simulink model "Robot_Leg_Kneel"  (R2025b)
settings: Solver=VariableStepAuto  StartTime=0.0  StopTime=20  RelTol=0.01  AbsTol=0.01  EnableMultiTasking=on
undefined symbols (not defined in the file): X, Y, Z
libraries: sm_lib x50, nesl_utility x37
(part 3 of 4)

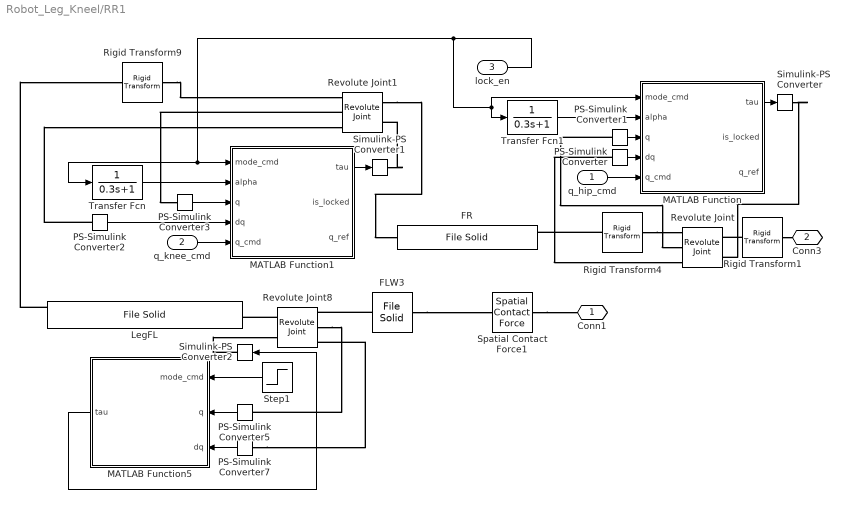
== system Robot_Leg_Kneel/RR1 ==
  q_hip_cmd : Inport
  q_knee_cmd : Inport  Port=2
  lock_en : Inport  Port=3
  FLW3 : sm_lib/Body Elements/File Solid  ExtGeomFileName=Cheng Shin C-166-1.stp  UnitType=FromFile  ExtGeomFileUnits=m  StepReaderType=HEX  ExportConvexHullGeometry=on  InertiaType=CalculateFromGeometry  BasedOnType=Density  Density=400  DensityUnits=kg/m^3  Mass=1  MassUnits=kg  CenterOfMass=[0 0 0]  CenterOfMassUnits=m  MomentsOfInertia=[1 1 1]  MomentsOfInertiaUnits=kg*m^2  ProductsOfInertia=[0 0 0]  ProductsOfInertiaUnits=kg*m^2  GraphicType=FromGeometry  MarkerShape=Sphere  MarkerSize=10  GraphicVisPropType=AdvancedVisualProperties  GraphicDiffuseColor=[0.1 0.1 0.1]  GraphicOpacity=1  GraphicSpecularColor=[0.2 0.2 0.2 1.0]  GraphicAmbientColor=[0.05 0.05 0.05 1.0]  GraphicEmissiveColor=[0.0 0.0 0.0 1.0]  GraphicShininess=10  DoExposeReferenceFrame=off  SerializedFrames=|
      | <Frames>
      | 
      |   <Frame>
      |     <Id>Frame1</Id>
      |     <Value>
      |       <Name>F1</Name>
      |       <Origin>
      |         <Source>GeometricFeature</Source>
      |         <FeatureName>toroidal surface 99</FeatureName>
      |       </Origin>
      |       <PrimaryAxis>
      |         <DefinedDirection>+Z</DefinedDirection>
      |         <Source>ReferenceFrame</Source>
      |         <SourceDirection>+Z</SourceDirection>
      |         <FeatureName></FeatureName>
      |       </PrimaryAxis>
      |       <SecondaryAxis>
      |         <DefinedDirection>+X</DefinedDirection>
      |         <Source>ReferenceFrame</Source>
      |         <SourceDirection>+X</SourceDirection>
      |         <FeatureName></FeatureName>
      |       </SecondaryAxis>
      |     </Value>
      |   </Frame>
      | 
      | </Frames>
  FR : sm_lib/Body Elements/File Solid  ExtGeomFileName=haut patte D.STEP  UnitType=FromFile  ExtGeomFileUnits=m  StepReaderType=HEX  ExportConvexHullGeometry=on  InertiaType=CalculateFromGeometry  BasedOnType=Density  Density=800  DensityUnits=kg/m^3  Mass=1  MassUnits=kg  CenterOfMass=[0 0 0]  CenterOfMassUnits=m  MomentsOfInertia=[1 1 1]  MomentsOfInertiaUnits=kg*m^2  ProductsOfInertia=[0 0 0]  ProductsOfInertiaUnits=kg*m^2  GraphicType=FromGeometry  MarkerShape=Sphere  MarkerSize=10  GraphicVisPropType=AdvancedVisualProperties  GraphicDiffuseColor=[0.9 0.9 0.9]  GraphicOpacity=1  GraphicSpecularColor=[0.9 0.9 0.9 1.0]  GraphicAmbientColor=[0.1 0.1 0.1 1.0]  GraphicEmissiveColor=[0.0 0.0 0.0 1.0]  GraphicShininess=100  DoExposeReferenceFrame=off  SerializedFrames=<Frames><Frame><Id>Frame1</Id><Value><Name>H-L link</Name><Origin><Source>GeometricFeature</Source><FeatureName>spherical surface 2</FeatureName></Origin><PrimaryAxis><DefinedDirection>+Z</DefinedDirection><Source>ReferenceFrame</Source><SourceDirection>+Z</SourceDirection><FeatureName></FeatureName></PrimaryAxis><SecondaryAxis><DefinedDirection>+X</DefinedDirection><Source>ReferenceFrame</Source><SourceDirection>-Y</SourceDirection><FeatureName></FeatureName></SecondaryAxis></Value></Frame><Frame><Id>Frame2</Id><Value><Name>L-K link</Name><Origin><Source>GeometricFeature</Source><FeatureName>cylindrical surface 2</FeatureName></Origin><PrimaryAxis><DefinedDirection>+Z</DefinedDirection><Source>ReferenceFrame</Source><SourceDirection>+Z</SourceDirection><FeatureName></FeatureName></PrimaryAxis><SecondaryAxis><DefinedDirection>+X</DefinedDirection><Source>ReferenceFrame</Source><SourceDirection>-Y</SourceDirection><FeatureName></FeatureName></SecondaryAxis></Value></Frame></Frames>
  LegFL : sm_lib/Body Elements/File Solid  ExtGeomFileName=leg.STEP  UnitType=FromFile  ExtGeomFileUnits=m  StepReaderType=HEX  ExportConvexHullGeometry=on  InertiaType=CalculateFromGeometry  BasedOnType=Density  Density=800  DensityUnits=kg/m^3  Mass=1  MassUnits=kg  CenterOfMass=[0 0 0]  CenterOfMassUnits=m  MomentsOfInertia=[1 1 1]  MomentsOfInertiaUnits=kg*m^2  ProductsOfInertia=[0 0 0]  ProductsOfInertiaUnits=kg*m^2  GraphicType=FromGeometry  MarkerShape=Sphere  MarkerSize=10  GraphicVisPropType=AdvancedVisualProperties  GraphicDiffuseColor=[0 0 0]  GraphicOpacity=1  GraphicSpecularColor=[0.9 0.9 0.9 1.0]  GraphicAmbientColor=[0.1 0.1 0.1 1.0]  GraphicEmissiveColor=[0.0 0.0 0.0 1.0]  GraphicShininess=100  DoExposeReferenceFrame=off  SerializedFrames=|
      | <Frames>
      | 
      |   <Frame>
      |     <Id>Frame1</Id>
      |     <Value>
      |       <Name>L-K link</Name>
      |       <Origin>
      |         <Source>GeometricFeature</Source>
      |         <FeatureName>cylindrical surface 6</FeatureName>
      |       </Origin>
      |       <PrimaryAxis>
      |         <DefinedDirection>+Z</DefinedDirection>
      |         <Source>ReferenceFrame</Source>
      |         <SourceDirection>+Z</SourceDirection>
      |         <FeatureName></FeatureName>
      |       </PrimaryAxis>
      |       <SecondaryAxis>
      |         <DefinedDirection>+X</DefinedDirection>
      |         <Source>ReferenceFrame</Source>
      |         <SourceDirection>-X</SourceDirection>
      |         <FeatureName></FeatureName>
      |       </SecondaryAxis>
      |     </Value>
      |   </Frame>
      | 
      |   <Frame>
      |     <Id>Frame2</Id>
      |     <Value>
      |       <Name>L-W link</Name>
      |       <Origin>
      |         <Source>GeometricFeature</Source>
      |         <FeatureName>cylindrical surface 4</FeatureName>
      |       </Origin>
      |       <PrimaryAxis>
      |         <DefinedDirection>+Z</DefinedDirection>
      |         <Source>ReferenceFrame</Source>
      |         <SourceDirection>+Z</SourceDirection>
      |         <FeatureName></FeatureName>
      |       </PrimaryAxis>
      |       <SecondaryAxis>
      |         <DefinedDirection>+X</DefinedDirection>
      |         <Source>ReferenceFrame</Source>
      |         <SourceDirection>-X</SourceDirection>
      |         <FeatureName></FeatureName>
      |       </SecondaryAxis>
      |     </Value>
      |   </Frame>
      | 
      | </Frames>
  MATLAB Function : MATLAB Function  TreatAsAtomicUnit=on  SystemSampleTime=0.002
  MATLAB Function1 : MATLAB Function  TreatAsAtomicUnit=on  SystemSampleTime=0.002
  MATLAB Function5 : MATLAB Function  TreatAsAtomicUnit=on
  PS-Simulink Converter{,1..3,5,7} (6 alike) : nesl_utility/PS-Simulink Converter  PhysicalDomain=network_engine_domain  SubClassName=ps_output  LeftPortType=input  RightPortType=output  PseudoPeriodic=off  Frequencies=[]  VectorFormat=inherit  Unit=inherit  AffineConversion=off
  Revolute Joint : sm_lib/Joints/Revolute Joint  JointMode=Normal  CompositeWrenchDir=FollowerOnBase  CompositeWrenchFrame=BaseFrame  SenseConstraintForce=off  SenseConstraintTorque=off  SenseTotalForce=off  SenseTotalTorque=off  PositionTargetSpecify=off  PositionTargetPriority=High  PositionTargetValue=0  PositionTargetValueUnits=deg  VelocityTargetSpecify=off  VelocityTargetPriority=High  VelocityTargetValue=0  VelocityTargetValueUnits=deg/s  EquilibriumPosition=0  EquilibriumPositionUnits=deg  SpringStiffness=0  SpringStiffnessUnits=N*m/deg  DampingCoefficient=0  DampingCoefficientUnits=N*m/(deg/s)  LowerLimitSpecify=off  LowerLimitBound=-90  LowerLimitBoundUnits=deg  LowerLimitStiffness=1e4  LowerLimitStiffnessUnits=N*m/deg  LowerLimitDamping=10  LowerLimitDampingUnits=N*m/(deg/s)  LowerLimitTransitionRegionWidth=0.1  LowerLimitTransitionRegionWidthUnits=deg  UpperLimitSpecify=off  UpperLimitBound=90  UpperLimitBoundUnits=deg  UpperLimitStiffness=1e4  UpperLimitStiffnessUnits=N*m/deg  UpperLimitDamping=10  UpperLimitDampingUnits=N*m/(deg/s)  UpperLimitTransitionRegionWidth=0.1  UpperLimitTransitionRegionWidthUnits=deg  TorqueActuationMode=InputTorque  MotionActuationMode=ComputedMotion  SensePosition=on  SenseVelocity=on  SenseAcceleration=off  SenseTorqueForce=off  SenseLowerLimitTorqueForce=off  SenseUpperLimitTorqueForce=off
  Revolute Joint1 : sm_lib/Joints/Revolute Joint  JointMode=Normal  CompositeWrenchDir=FollowerOnBase  CompositeWrenchFrame=BaseFrame  SenseConstraintForce=off  SenseConstraintTorque=off  SenseTotalForce=off  SenseTotalTorque=off  PositionTargetSpecify=off  PositionTargetPriority=High  PositionTargetValue=0  PositionTargetValueUnits=deg  VelocityTargetSpecify=off  VelocityTargetPriority=High  VelocityTargetValue=0  VelocityTargetValueUnits=deg/s  EquilibriumPosition=0  EquilibriumPositionUnits=deg  SpringStiffness=0  SpringStiffnessUnits=N*m/deg  DampingCoefficient=0  DampingCoefficientUnits=N*m/(deg/s)  LowerLimitSpecify=off  LowerLimitBound=-90  LowerLimitBoundUnits=deg  LowerLimitStiffness=1e4  LowerLimitStiffnessUnits=N*m/deg  LowerLimitDamping=10  LowerLimitDampingUnits=N*m/(deg/s)  LowerLimitTransitionRegionWidth=0.1  LowerLimitTransitionRegionWidthUnits=deg  UpperLimitSpecify=off  UpperLimitBound=90  UpperLimitBoundUnits=deg  UpperLimitStiffness=1e4  UpperLimitStiffnessUnits=N*m/deg  UpperLimitDamping=10  UpperLimitDampingUnits=N*m/(deg/s)  UpperLimitTransitionRegionWidth=0.1  UpperLimitTransitionRegionWidthUnits=deg  TorqueActuationMode=InputTorque  MotionActuationMode=ComputedMotion  SensePosition=on  SenseVelocity=on  SenseAcceleration=off  SenseTorqueForce=off  SenseLowerLimitTorqueForce=off  SenseUpperLimitTorqueForce=off
  Revolute Joint8 : sm_lib/Joints/Revolute Joint  JointMode=Normal  CompositeWrenchDir=FollowerOnBase  CompositeWrenchFrame=BaseFrame  SenseConstraintForce=off  SenseConstraintTorque=off  SenseTotalForce=off  SenseTotalTorque=off  PositionTargetSpecify=off  PositionTargetPriority=High  PositionTargetValue=0  PositionTargetValueUnits=deg  VelocityTargetSpecify=off  VelocityTargetPriority=High  VelocityTargetValue=0  VelocityTargetValueUnits=deg/s  EquilibriumPosition=0  EquilibriumPositionUnits=deg  SpringStiffness=0  SpringStiffnessUnits=N*m/deg  DampingCoefficient=0  DampingCoefficientUnits=N*m/(deg/s)  LowerLimitSpecify=off  LowerLimitBound=-90  LowerLimitBoundUnits=deg  LowerLimitStiffness=1e4  LowerLimitStiffnessUnits=N*m/deg  LowerLimitDamping=10  LowerLimitDampingUnits=N*m/(deg/s)  LowerLimitTransitionRegionWidth=0.1  LowerLimitTransitionRegionWidthUnits=deg  UpperLimitSpecify=off  UpperLimitBound=90  UpperLimitBoundUnits=deg  UpperLimitStiffness=1e4  UpperLimitStiffnessUnits=N*m/deg  UpperLimitDamping=10  UpperLimitDampingUnits=N*m/(deg/s)  UpperLimitTransitionRegionWidth=0.1  UpperLimitTransitionRegionWidthUnits=deg  TorqueActuationMode=InputTorque  MotionActuationMode=ComputedMotion  SensePosition=on  SenseVelocity=on  SenseAcceleration=off  SenseTorqueForce=off  SenseLowerLimitTorqueForce=off  SenseUpperLimitTorqueForce=off
  Rigid Transform1 : sm_lib/Frames and Transforms/Rigid Transform  RotationMethod=AlignedAxes  FollAlignAxisA=+Z  BaseAlignAxisA=+Y  FollAlignAxisB=+X  BaseAlignAxisB=+X  RotationStandardAxis=+Z  RotationAngle=0  RotationAngleUnits=deg  RotationArbitraryAxis=[0 0 1]  RotationSequenceAxes=FollowerAxes  RotationSequence=XYX  RotationSequenceAngles=[0 0 0]  RotationSequenceAnglesUnits=deg  RotationMatrix=[1 0 0;0 1 0;0 0 1]  Quaternion=[1 0 0 0]  TranslationMethod=None  TranslationCartesianOffset=[0 0 0]  TranslationCartesianOffsetUnits=m  TranslationStandardAxis=+Z  TranslationStandardOffset=0  TranslationStandardOffsetUnits=m  TranslationROffset=0  TranslationROffsetUnits=m  TranslationThetaOffset=0  TranslationThetaOffsetUnits=deg  TranslationZOffset=0  TranslationZOffsetUnits=m
  Rigid Transform4 : sm_lib/Frames and Transforms/Rigid Transform  RotationMethod=RotationSequence  FollAlignAxisA=+X  BaseAlignAxisA=+Y  FollAlignAxisB=+Y  BaseAlignAxisB=+Z  RotationStandardAxis=+Z  RotationAngle=0  RotationAngleUnits=deg  RotationArbitraryAxis=[0 0 1]  RotationSequenceAxes=FollowerAxes  RotationSequence=XYZ  RotationSequenceAngles=[0 0 30]  RotationSequenceAnglesUnits=deg  RotationMatrix=[1 0 0;0 1 0;0 0 1]  Quaternion=[1 0 0 0]  TranslationMethod=None  TranslationCartesianOffset=[0 0 0]  TranslationCartesianOffsetUnits=m  TranslationStandardAxis=+Z  TranslationStandardOffset=0  TranslationStandardOffsetUnits=m  TranslationROffset=0  TranslationROffsetUnits=m  TranslationThetaOffset=0  TranslationThetaOffsetUnits=deg  TranslationZOffset=0  TranslationZOffsetUnits=m
  Rigid Transform9 : sm_lib/Frames and Transforms/Rigid Transform  RotationMethod=RotationSequence  FollAlignAxisA=+X  BaseAlignAxisA=+Y  FollAlignAxisB=+Y  BaseAlignAxisB=+Z  RotationStandardAxis=+Z  RotationAngle=0  RotationAngleUnits=deg  RotationArbitraryAxis=[0 0 1]  RotationSequenceAxes=FollowerAxes  RotationSequence=XYZ  RotationSequenceAngles=[0 0 -30]  RotationSequenceAnglesUnits=deg  RotationMatrix=[1 0 0;0 1 0;0 0 1]  Quaternion=[1 0 0 0]  TranslationMethod=None  TranslationCartesianOffset=[0 0 0]  TranslationCartesianOffsetUnits=m  TranslationStandardAxis=+Z  TranslationStandardOffset=0  TranslationStandardOffsetUnits=m  TranslationROffset=0  TranslationROffsetUnits=m  TranslationThetaOffset=0  TranslationThetaOffsetUnits=deg  TranslationZOffset=0  TranslationZOffsetUnits=m
  Simulink-PS Converter : nesl_utility/Simulink-PS Converter  PhysicalDomain=network_engine_domain  SubClassName=ps_input  LeftPortType=input  RightPortType=output  PseudoPeriodic=off  Frequencies=[]  NoiseDistribution=none  NoiseParameters=[]  Unit=1  AffineConversion=off  FilteringAndDerivatives=provide  SimscapeFilterOrder=1  InputFilterTimeConstant=0.001  UdotUserProvided=0
  Simulink-PS Converter1 : nesl_utility/Simulink-PS Converter  PhysicalDomain=network_engine_domain  SubClassName=ps_input  LeftPortType=input  RightPortType=output  PseudoPeriodic=off  Frequencies=[]  NoiseDistribution=none  NoiseParameters=[]  Unit=1  AffineConversion=off  FilteringAndDerivatives=provide  SimscapeFilterOrder=1  InputFilterTimeConstant=0.001  UdotUserProvided=0
  Simulink-PS Converter2 : nesl_utility/Simulink-PS Converter  PhysicalDomain=network_engine_domain  SubClassName=ps_input  LeftPortType=input  RightPortType=output  PseudoPeriodic=off  Frequencies=[]  NoiseDistribution=none  NoiseParameters=[]  Unit=1  AffineConversion=off  FilteringAndDerivatives=provide  SimscapeFilterOrder=1  InputFilterTimeConstant=0.001  UdotUserProvided=0
  Spatial Contact Force1 : sm_lib/Forces and Torques/Spatial Contact Force  SenseSeparationDistance=off  NormalForceType=SmoothSpringDamper  NormalStiffness=1e6  NormalStiffnessUnits=N/m  NormalDamping=1e3  NormalDampingUnits=N/(m/s)  NormalTransitionRegionWidth=1e-4  NormalTransitionRegionWidthUnits=m  FrictionType=SmoothStickSlip  CoefficientOfStaticFriction=0.9  CoefficientOfDynamicFriction=0.7  FrictionalCriticalVelocity=1e-3  FrictionalCriticalVelocityUnits=m/s  SenseContactSignal=off  SensePenetrationDepth=off  SenseNormalVelocity=off  SenseTangentialVelocity=off  SensingForceTorqueDirection=BaseOnFollower  SensingForceTorqueResolutionFrame=ContactFrame  SenseNormalForce=off  SenseNormalForceMagnitude=off  SenseNormalTorque=off  SenseFrictionalForce=off  SenseFrictionalForceMagnitude=off  SenseFrictionalTorque=off  SenseTotalForce=off  SenseTotalTorque=off  SenseContactBaseRotation=off  SenseContactBaseTranslation=off  SenseContactFollowerRotation=off  SenseContactFollowerTranslation=off  ZeroCrossDetectContactStartAndEnd=off
  Step1 : Step  Time=3  Before=1  After=0  SampleTime=0
  Transfer Fcn : TransferFcn  Denominator=[0.3 1]
  Transfer Fcn1 : TransferFcn  Denominator=[0.3 1]
  Conn1 : PMIOPort  Side=Left
  Conn3 : PMIOPort  Port=2  Side=Right
  wires:
  MATLAB Function/1(tau) -> Simulink-PS Converter/1
  PS-Simulink Converter3/1 -> MATLAB Function1/3(q)
  lock_en/1 -> MATLAB Function/1(mode_cmd), Transfer Fcn1/1, Transfer Fcn/1, MATLAB Function1/1(mode_cmd)
  PS-Simulink Converter2/1 -> MATLAB Function1/4(dq)
  PS-Simulink Converter/1 -> MATLAB Function/4(dq)
  PS-Simulink Converter1/1 -> MATLAB Function/3(q)
  MATLAB Function1/1(tau) -> Simulink-PS Converter1/1
  Transfer Fcn1/1 -> MATLAB Function/2(alpha)
  q_knee_cmd/1 -> MATLAB Function1/5(q_cmd)
  q_hip_cmd/1 -> MATLAB Function/5(q_cmd)
  MATLAB Function5/1(tau) -> Simulink-PS Converter2/1
  Transfer Fcn/1 -> MATLAB Function1/2(alpha)
  Step1/1 -> MATLAB Function5/1(mode_cmd)
  PS-Simulink Converter7/1 -> MATLAB Function5/3(dq)
  PS-Simulink Converter5/1 -> MATLAB Function5/2(q)
  connections:
  Rigid Transform1/RConn1 -- Revolute Joint/LConn1
  Simulink-PS Converter1/RConn1 -- Revolute Joint1/LConn2
  Revolute Joint8/LConn1 -- LegFL/RConn1
  Rigid Transform4/LConn1 -- Revolute Joint/RConn1
  PS-Simulink Converter2/LConn1 -- Revolute Joint1/RConn3
  PS-Simulink Converter/LConn1 -- Revolute Joint/RConn3
  Revolute Joint1/RConn2 -- PS-Simulink Converter3/LConn1
  Simulink-PS Converter/RConn1 -- Revolute Joint/LConn2
  PS-Simulink Converter1/LConn1 -- Revolute Joint/RConn2
  Rigid Transform1/LConn1 -- Conn3/RConn1
  Simulink-PS Converter2/RConn1 -- Revolute Joint8/LConn2
  Spatial Contact Force1/LConn1 -- Conn1/RConn1
  FLW3/LConn1 -- Revolute Joint8/RConn1
  FLW3/RConn1 -- Spatial Contact Force1/RConn1
  Rigid Transform4/RConn1 -- FR/LConn1
  Revolute Joint1/LConn1 -- FR/RConn1
  Rigid Transform9/LConn1 -- Revolute Joint1/RConn1
  LegFL/LConn1 -- Rigid Transform9/RConn1
  Revolute Joint8/RConn2 -- PS-Simulink Converter5/LConn1
  PS-Simulink Converter7/LConn1 -- Revolute Joint8/RConn3

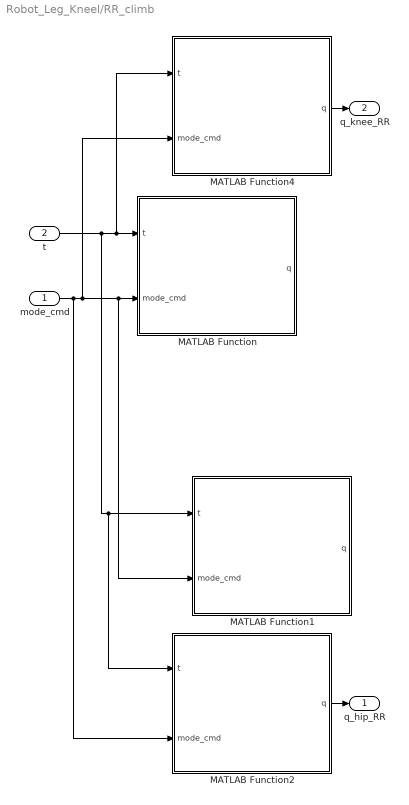
== system Robot_Leg_Kneel/RR_climb ==
  mode_cmd : Inport
  t : Inport  Port=2
  MATLAB Function : MATLAB Function  TreatAsAtomicUnit=on
  MATLAB Function1 : MATLAB Function  TreatAsAtomicUnit=on
  MATLAB Function2 : MATLAB Function  TreatAsAtomicUnit=on
  MATLAB Function4 : MATLAB Function  TreatAsAtomicUnit=on
  q_hip_RR : Outport
  q_knee_RR : Outport  Port=2
  wires:
  t/1 -> MATLAB Function2/1(t), MATLAB Function1/1(t), MATLAB Function4/1(t), MATLAB Function/1(t)
  mode_cmd/1 -> MATLAB Function2/2(mode_cmd), MATLAB Function4/2(mode_cmd), MATLAB Function1/2(mode_cmd), MATLAB Function/2(mode_cmd)
  MATLAB Function2/1(q) -> q_hip_RR/1
  MATLAB Function4/1(q) -> q_knee_RR/1

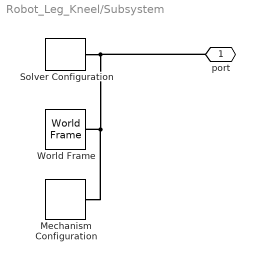
== system Robot_Leg_Kneel/Subsystem ==
  Mechanism Configuration : sm_lib/Utilities/Mechanism Configuration  UniformGravity=Constant  GravityVector=[0 0 -9.80665]  GravityVectorUnits=m/s^2  LinearizationDelta=0.001  JointModeTransitionNonlinearIterations=2
  Solver Configuration : nesl_utility/Solver Configuration  PhysicalDomain=network_engine_domain  SubClassName=solver  LeftPortType=input  RightPortType=generic  Tones=[]  Harmonics=[]  SimulateNoise=off  Profile=off  UseLocalSampling=off  EnableSwitchedLinearOptims=on  FrequencyDomain=off  UseCCode=off  RelTol=0.001  AbsTol=1e-06  MinStep=1e-09  ToWorkspace=off  RevertToSquareIcSolve=off  NumHomotopyIterations=100  PhasorMode=off  PhasorModeNumHarmonics=1  ConsistencySolver=NEWTON_XTOL_AFTER_FTOL  IndexReductionMethod=DerivativeReplacement  DoDC=off  ResidualTolerance=1e-09  ConsistencyTolSource=GLOBAL  ConsistencyAbsTol=0.001  ConsistencyRelTol=0.001  ConsistencyTolFactor=0.001  UseLocalSolver=off  LocalSolverChoice=NE_BACKWARD_EULER_ADVANCER  ResolveIndetEquations=on  FunctionEvalNumThread=1  LocalSolverSampleTime=0.001  DoFixedCost=off  MaxNonlinIter=3  MaxModeIter=2  ComputeImpulses=off  ImpulseIterations=2  LinearAlgebra=Sparse  LinearAlgebraNumThread=0  EquationFormulation=NE_TIME_EF  DelaysMemoryBudget=1024  AutomaticFiltering=on  FilteringTimeConstant=0.001  PartitionStorageMethod=AS_NEEDED  PartitionMemoryBudget=1024  PartitionMethod=FAST  MultibodyUseLocalSolver=off  MultibodyLocalSolverChoice=ODE1  MultibodyLocalSolverSampleTime=0.001
  World Frame : sm_lib/Frames and Transforms/World Frame
  port : PMIOPort  Side=Right
  connections:
  Solver Configuration/RConn1 -- port/RConn1 -- Mechanism Configuration/RConn1 -- World Frame/RConn1

== matlab function Robot_Leg_Kneel/RL/MATLAB Function1 ==
  data: mode_cmd input; alpha input; tau output; q input; dq input; q_cmd input; is_locked output; q_ref output
function [tau, is_locked, q_ref] = LockJointPD(mode_cmd, alpha, q, dq, q_cmd)
%#codegen
% mode_cmd: 0=Walk (track q_cmd), 1=Wheeled (lock current angle)
% alpha   : [0,1] smoothing factor (TransferFcn output), 0=fully walking, 1=fully locked
% q,dq    : joint angle/angular velocity
% q_cmd   : walk/stand target angle (radians)
Kp = 1200.0;   % Starting value, tune per joint
Kd =   20.0;
tau_lim = 300.0;
m = uint8(mode_cmd ~= 0);     % Standardize to uint8(0/1)
a = double(alpha);
persistent q_hold last_mode
if isempty(q_hold),    q_hold    = q;        end   % double
if isempty(last_mode), last_mode = uint8(0); end   % uint8
% Rising edge: 0->1, latch current angle
if (last_mode == uint8(0)) && (m ~= uint8(0))
    q_hold = q;
end
last_mode = m;
% Reference angle: interpolate between "hold angle" and "target angle"
q_ref  = a*q_hold + (1-a)*q_cmd;
dq_ref = 0.0;
% PD
tau = Kp*(q_ref - q) + Kd*(dq_ref - dq);
% Saturation
tau = max(min(tau, tau_lim), -tau_lim);
% Debug flag: is leg lock dominant
is_locked = (a > 0.5);     % Can also output m==1
end

== matlab function Robot_Leg_Kneel/RL1/MATLAB Function5 ==
  settings: updateMethod=DISCRETE
  data: mode_cmd input; tau output; q input; dq input
function tau = WheelLockPD(mode_cmd, q, dq)
%#codegen
% mode_cmd: 0=Walk (lock wheel), 1=Wheeled (don't lock wheel)
% q, dq measurements from the wheel axle Revolute Joint
% Braking PD parameters (tunable)
Kp = 50.0;     % Braking stiffness, smaller to avoid being too rigid
Kd =  5.0;     % Damping
tau_lim = 150.0;  % Maximum braking torque for the wheel
% Lock only in walk mode
lock = (mode_cmd == 0);
persistent q_hold last_lock
if isempty(q_hold),    q_hold    = q;     end
if isempty(last_lock), last_lock = false; end
% The moment it switches from "unlocked" to "locked", remember the current angle
if (~last_lock) && lock
    q_hold = q;
end
last_lock = lock;
if lock
    % Lock wheel: treat q_hold as the target angle
    q_ref  = q_hold;
    dq_ref = 0.0;
    tau = Kp*(q_ref - q) + Kd*(dq_ref - dq);
else
    % Wheeled mode: do not apply brake
    tau = 0.0;
end
% Torque saturation
if tau >  tau_lim, tau =  tau_lim; end
if tau < -tau_lim, tau = -tau_lim; end
end

== matlab function Robot_Leg_Kneel/RR1/MATLAB Function5 ==
  settings: updateMethod=DISCRETE
  data: mode_cmd input; tau output; q input; dq input
function tau = WheelLockPD(mode_cmd, q, dq)
%#codegen
% mode_cmd: 0=Walk (lock wheel), 1=Wheeled (don't lock wheel)
% q, dq measurements from the wheel axle Revolute Joint
% Braking PD parameters (tunable)
Kp = 50.0;     % Braking stiffness, smaller to avoid being too rigid
Kd =  5.0;     % Damping
tau_lim = 150.0;  % Maximum braking torque for the wheel
% Lock only in walk mode
lock = (mode_cmd == 0);
persistent q_hold last_lock
if isempty(q_hold),    q_hold    = q;     end
if isempty(last_lock), last_lock = false; end
% The moment it switches from "unlocked" to "locked", remember the current angle
if (~last_lock) && lock
    q_hold = q;
end
last_lock = lock;
if lock
    % Lock wheel: treat q_hold as the target angle
    q_ref  = q_hold;
    dq_ref = 0.0;
    tau = Kp*(q_ref - q) + Kd*(dq_ref - dq);
else
    % Wheeled mode: do not apply brake
    tau = 0.0;
end
% Torque saturation
if tau >  tau_lim, tau =  tau_lim; end
if tau < -tau_lim, tau = -tau_lim; end
end

== matlab function Robot_Leg_Kneel/RR_climb/MATLAB Function ==
  data: t input; q output; mode_cmd input
function q = knee_FL_motion(t, mode_cmd)
%#codegen

Tsw = 102;   % 切换时间

% ------- 轮式模式：锁住，腿不动 -------
if (mode_cmd == 1) || (t < Tsw)
    q = 0;          % 回到原位（站立角）
    return;
end

% ------- 腿式模式：先蹲再站 -------
tau = t - Tsw;      % 本地时间

% 对应髋关节的三个阶段：T1 蹲下，T2 保持，T3 站起
T1 = 3;    % 蹲下用时
T2 = 15;    % 低姿态保持时间
T3 = 3;    % 站起用时

% 膝关节的站立角和蹲下角
q_stand = 0;                % 站立时膝盖角（回原位就是这个）
q_squat = -deg2rad(70);      % 蹲下时膝盖最大弯曲

% --- 段1：从站立 -> 蹲下 ---
if tau < T1
    u = tau / T1;                           % 0→1
    q = (1-u)*q_stand + u*q_squat;

% --- 段2：保持蹲下姿态 ---
elseif tau < T1 + T2
    q = q_squat;

% --- 段3：从蹲下 -> 回到原位 ---
elseif tau < T1 + T2 + T3
    u = (tau - (T1 + T2)) / T3;
    q = (1-u)*q_squat + u*q_stand;

% --- 结束后一直保持原位 ---
else
    q = q_stand;
end
end

== matlab function Robot_Leg_Kneel/FR_climb/MATLAB Function2 ==
  data: t input; q output; mode_cmd input
function q = knee_FL_motion(t, mode_cmd)
%#codegen

Tsw = 102;   % 切换时间

% ------- 轮式模式：锁住，腿不动 -------
if (mode_cmd == 1) || (t < Tsw)
    q = 0;          % 回到原位（站立角）
    return;
end

% ------- 腿式模式：先蹲再站 -------
tau = t - Tsw;      % 本地时间

% 对应髋关节的三个阶段：T1 蹲下，T2 保持，T3 站起
T1 = 3;    % 蹲下用时
T2 = 15;    % 低姿态保持时间
T3 = 3;    % 站起用时

% 膝关节的站立角和蹲下角
q_stand = 0;                % 站立时膝盖角（回原位就是这个）
q_squat = -deg2rad(70);      % 蹲下时膝盖最大弯曲

% --- 段1：从站立 -> 蹲下 ---
if tau < T1
    u = tau / T1;                           % 0→1
    q = (1-u)*q_stand + u*q_squat;

% --- 段2：保持蹲下姿态 ---
elseif tau < T1 + T2
    q = q_squat;

% --- 段3：从蹲下 -> 回到原位 ---
elseif tau < T1 + T2 + T3
    u = (tau - (T1 + T2)) / T3;
    q = (1-u)*q_squat + u*q_stand;

% --- 结束后一直保持原位 ---
else
    q = q_stand;
end
end

== matlab function Robot_Leg_Kneel/RL_climb/MATLAB Function ==
  data: t input; q output; mode_cmd input
function q = knee_FL_motion(t, mode_cmd)
%#codegen

Tsw = 102;   % 切换时间

% ------- 轮式模式：锁住，腿不动 -------
if (mode_cmd == 1) || (t < Tsw)
    q = 0;          % 回到原位（站立角）
    return;
end

% ------- 腿式模式：先蹲再站 -------
tau = t - Tsw;      % 本地时间

% 对应髋关节的三个阶段：T1 蹲下，T2 保持，T3 站起
T1 = 3;    % 蹲下用时
T2 = 15;    % 低姿态保持时间
T3 = 3;    % 站起用时

% 膝关节的站立角和蹲下角
q_stand = 0;                % 站立时膝盖角（回原位就是这个）
q_squat = -deg2rad(70);      % 蹲下时膝盖最大弯曲

% --- 段1：从站立 -> 蹲下 ---
if tau < T1
    u = tau / T1;                           % 0→1
    q = (1-u)*q_stand + u*q_squat;

% --- 段2：保持蹲下姿态 ---
elseif tau < T1 + T2
    q = q_squat;

% --- 段3：从蹲下 -> 回到原位 ---
elseif tau < T1 + T2 + T3
    u = (tau - (T1 + T2)) / T3;
    q = (1-u)*q_squat + u*q_stand;

% --- 结束后一直保持原位 ---
else
    q = q_stand;
end
end

== matlab function Robot_Leg_Kneel/FL_climb/MATLAB Function2 ==
  data: t input; q output; mode_cmd input
function q = hip_FL_motion(t, mode_cmd)
%#codegen
% --- 左前腿 (Front Left) 髋关节 ---
% 策略：锁轮爬梯。先迈步，然后负责拉动身体前移。

T_squat_start = 5;
T_climb_start = 30;

% --- 阶段 0: 轮式/未开始 ---
if (mode_cmd == 1) || (t < T_squat_start); q = 0; return; end

% --- 阶段 1: 原地蹲起测试 (102s-130s) ---
if t < T_climb_start
    tau = t - T_squat_start;
    q_stand = 0; q_squat = deg2rad(35);
    T1 = 3; T2 = 5; T3 = 3;
    if tau < T1; u=tau/T1; q=(1-u)*q_stand+u*q_squat;
    elseif tau < T1+T2; q=q_squat;
    elseif tau < T1+T2+T3; u=(tau-(T1+T2))/T3; q=(1-u)*q_squat+u*q_stand;
    else; q=q_stand; end
    return;
end

% ==========================================
% 阶段 2: 锁轮爬台阶 (130s 开始)
% ==========================================
tau = t - T_climb_start;

% 参数 (小步幅)
    q_neutral = 0;
    q_fwd     = deg2rad(-5); % 往前伸
    
    % [130-132] 第一步：抬腿迈向前方
    if tau < 2.0
        u = tau / 2.0;
        q = (1-u)*q_neutral + u*q_fwd;
        
    % [132-134] 等待右前腿 (保持在前)
    elseif tau < 4.0
        q = q_fwd;
        
    % [134-138] 全身前移 (Body Shift)
    % 关键：此时腿是着地的，Hip从"前"转回"中立"，相当于把身体拉过去
    elseif tau < 8.0
        dt = tau - 4.0;
        u = dt / 4.0; % 给4秒慢慢拉，防止前轮打滑
        u_smooth = 0.5 * (1 - cos(u * pi));
        q = (1-u_smooth)*q_fwd + u_smooth*q_neutral;
        
    % [138+] 动作完成，保持中立
    else
        q = q_neutral;
    end
end

== matlab function Robot_Leg_Kneel/RR/MATLAB Function1 ==
  data: mode_cmd input; alpha input; tau output; q input; dq input; q_cmd input; is_locked output; q_ref output
function [tau, is_locked, q_ref] = LockJointPD(mode_cmd, alpha, q, dq, q_cmd)
%#codegen
% mode_cmd: 0=Walk (track q_cmd), 1=Wheeled (lock current angle)
% alpha   : [0,1] smoothing factor (TransferFcn output), 0=fully walking, 1=fully locked
% q,dq    : joint angle/angular velocity
% q_cmd   : walk/stand target angle (radians)
Kp = 1200.0;   % Starting value, tune per joint
Kd =   20.0;
tau_lim = 300.0;
m = uint8(mode_cmd ~= 0);     % Standardize to uint8(0/1)
a = double(alpha);
persistent q_hold last_mode
if isempty(q_hold),    q_hold    = q;        end   % double
if isempty(last_mode), last_mode = uint8(0); end   % uint8
% Rising edge: 0->1, latch current angle
if (last_mode == uint8(0)) && (m ~= uint8(0))
    q_hold = q;
end
last_mode = m;
% Reference angle: interpolate between "hold angle" and "target angle"
q_ref  = a*q_hold + (1-a)*q_cmd;
dq_ref = 0.0;
% PD
tau = Kp*(q_ref - q) + Kd*(dq_ref - dq);
% Saturation
tau = max(min(tau, tau_lim), -tau_lim);
% Debug flag: is leg lock dominant
is_locked = (a > 0.5);     % Can also output m==1
end

== matlab function Robot_Leg_Kneel/FL_climb/MATLAB Function1 ==
  data: t input; q output; mode_cmd input
function q = knee_FL_motion(t, mode_cmd)
%#codegen

Tsw = 102;   % 切换时间

% ------- 轮式模式：锁住，腿不动 -------
if (mode_cmd == 1) || (t < Tsw)
    q = 0;          % 回到原位（站立角）
    return;
end

% ------- 腿式模式：先蹲再站 -------
tau = t - Tsw;      % 本地时间

% 对应髋关节的三个阶段：T1 蹲下，T2 保持，T3 站起
T1 = 3;    % 蹲下用时
T2 = 15;    % 低姿态保持时间
T3 = 3;    % 站起用时

% 膝关节的站立角和蹲下角
q_stand = 0;                % 站立时膝盖角（回原位就是这个）
q_squat = -deg2rad(70);      % 蹲下时膝盖最大弯曲

% --- 段1：从站立 -> 蹲下 ---
if tau < T1
    u = tau / T1;                           % 0→1
    q = (1-u)*q_stand + u*q_squat;

% --- 段2：保持蹲下姿态 ---
elseif tau < T1 + T2
    q = q_squat;

% --- 段3：从蹲下 -> 回到原位 ---
elseif tau < T1 + T2 + T3
    u = (tau - (T1 + T2)) / T3;
    q = (1-u)*q_squat + u*q_stand;

% --- 结束后一直保持原位 ---
else
    q = q_stand;
end
end

== matlab function Robot_Leg_Kneel/FL_climb/MATLAB Function3 ==
  data: t input; q output; mode_cmd input
function q = knee_FL_motion(t, mode_cmd)
%#codegen
% --- 左前腿 (Front Left) 膝关节 ---

T_squat_start = 5;
T_climb_start = 30;

% --- 阶段 0 & 1 ---
if (mode_cmd == 1) || (t < T_squat_start); q = 0; return; end
if t < T_climb_start
    tau = t - T_squat_start;
    q_stand = 0; q_squat = -deg2rad(70);
    T1 = 3; T2 = 5; T3 = 3;
    if tau < T1; u=tau/T1; q=(1-u)*q_stand+u*q_squat;
    elseif tau < T1+T2; q=q_squat;
    elseif tau < T1+T2+T3; u=(tau-(T1+T2))/T3; q=(1-u)*q_squat+u*q_stand;
    else; q=q_stand; end
    return;
end

% ==========================================
% 阶段 2: 锁轮爬台阶 (130s 开始)
% ==========================================
 tau = t - T_climb_start;
% --- 膝盖参数 ---
q_stand = deg2rad(0); % 站立微屈
    q_lift  = deg2rad(-20); % 小幅度抬腿
    
    % [130-132] 抬腿迈步
    if tau < 2.0
        u = tau / 2.0;
        lift_scale = sin(u * pi); 
        q = q_stand + lift_scale * (q_lift - q_stand);
        
    % [132+] 之后一直踩在地上用力
    else
        q = q_stand;
    end
end

== matlab function Robot_Leg_Kneel/FR_climb/MATLAB Function3 ==
  data: t input; q output; mode_cmd input
function q = hip_FL_motion(t, mode_cmd)
%#codegen

Tsw = 102;

% 轮式阶段：髋关节锁在 0
if (mode_cmd == 1) || (t < Tsw)
    q = 0;          % 轮式时锁住髋关节
    return;
end

% 腿式阶段：开始做“先蹲后站”的动作
tau = t - Tsw;      % 本地时间，从切换时刻重新计

% 姿态角（单位：rad）
q_stand = 0;                  % 站立时髋角
q_squat = deg2rad(35);       % 蹲下时髋角（负是往上收腿）
% 你觉得不够矮可以再调大一点绝对值，比如 -45°

% 时间设置（和膝盖可以对应着来）
T1 = 3;    % 蹲下用时
T2 = 15;    % 低姿态保持时间
T3 = 3;    % 站起来用时
% 总时长 T1+T2+T3 之后保持站立

% --- 段1：从站立 -> 蹲下 ---
if tau < T1
    u = tau / T1;                      % 0→1
    q = (1-u)*q_stand + u*q_squat;

% --- 段2：保持蹲下姿态 ---
elseif tau < T1 + T2
    q = q_squat;

% --- 段3：从蹲下 -> 站回原位 ---
elseif tau < T1 + T2 + T3
    u = (tau - (T1 + T2)) / T3;
    q = (1-u)*q_squat + u*q_stand;

% --- 结束后：保持站立 ---
else
    q = q_stand;
end
end

== matlab function Robot_Leg_Kneel/RL_climb/MATLAB Function1 ==
  data: t input; mode_cmd input; q output
function q= hip_FL_motion(t, mode_cmd)
%#codegen

Tsw = 102;

% 轮式阶段：髋关节锁在 0
if (mode_cmd == 1) || (t < Tsw)
    q = 0;          % 轮式时锁住髋关节
    return;
end

% 腿式阶段：开始做“先蹲后站”的动作
tau = t - Tsw;      % 本地时间，从切换时刻重新计

% 姿态角（单位：rad）
q_stand = 0;                  % 站立时髋角
q_squat = deg2rad(35);       % 蹲下时髋角（负是往上收腿）
% 你觉得不够矮可以再调大一点绝对值，比如 -45°

% 时间设置（和膝盖可以对应着来）
T1 = 3;    % 蹲下用时
T2 = 15;    % 低姿态保持时间
T3 = 3;    % 站起来用时
% 总时长 T1+T2+T3 之后保持站立

% --- 段1：从站立 -> 蹲下 ---
if tau < T1
    u = tau / T1;                      % 0→1
    q = (1-u)*q_stand + u*q_squat;

% --- 段2：保持蹲下姿态 ---
elseif tau < T1 + T2
    q = q_squat;

% --- 段3：从蹲下 -> 站回原位 ---
elseif tau < T1 + T2 + T3
    u = (tau - (T1 + T2)) / T3;
    q = (1-u)*q_squat + u*q_stand;

% --- 结束后：保持站立 ---
else
    q = q_stand;
end
end

== matlab function Robot_Leg_Kneel/RR_climb/MATLAB Function1 ==
  data: t input; q output; mode_cmd input
function q = hip_FL_motion(t, mode_cmd)
%#codegen

Tsw = 102;

% 轮式阶段：髋关节锁在 0
if (mode_cmd == 1) || (t < Tsw)
    q = 0;          % 轮式时锁住髋关节
    return;
end

% 腿式阶段：开始做“先蹲后站”的动作
tau = t - Tsw;      % 本地时间，从切换时刻重新计

% 姿态角（单位：rad）
q_stand = 0;                  % 站立时髋角
q_squat = deg2rad(35);       % 蹲下时髋角（负是往上收腿）

% 时间设置（和膝盖可以对应着来）
T1 = 3;    % 蹲下用时
T2 = 15;    % 低姿态保持时间
T3 = 3;    % 站起来用时
% 总时长 T1+T2+T3 之后保持站立

% --- 段1：从站立 -> 蹲下 ---
if tau < T1
    u = tau / T1;                      % 0→1
    q = (1-u)*q_stand + u*q_squat;

% --- 段2：保持蹲下姿态 ---
elseif tau < T1 + T2
    q = q_squat;

% --- 段3：从蹲下 -> 站回原位 ---
elseif tau < T1 + T2 + T3
    u = (tau - (T1 + T2)) / T3;
    q = (1-u)*q_squat + u*q_stand;

% --- 结束后：保持站立 ---
else
    q = q_stand;
end
end

== matlab function Robot_Leg_Kneel/FL_climb/MATLAB Function4 ==
  data: t input; q output; mode_cmd input
function q = hip_FL_motion(t, mode_cmd)
%#codegen

Tsw = 102;

% 轮式阶段：髋关节锁在 0
if (mode_cmd == 1) || (t < Tsw)
    q = 0;          % 轮式时锁住髋关节
    return;
end

% 腿式阶段：开始做“先蹲后站”的动作
tau = t - Tsw;      % 本地时间，从切换时刻重新计

% 姿态角（单位：rad）
q_stand = 0;                  % 站立时髋角
q_squat = deg2rad(35);       % 蹲下时髋角（负是往上收腿）

% 时间设置（和膝盖可以对应着来）
T1 = 3;    % 蹲下用时
T2 = 15;    % 低姿态保持时间
T3 = 3;    % 站起来用时
% 总时长 T1+T2+T3 之后保持站立

% --- 段1：从站立 -> 蹲下 ---
if tau < T1
    u = tau / T1;                      % 0→1
    q = (1-u)*q_stand + u*q_squat;

% --- 段2：保持蹲下姿态 ---
elseif tau < T1 + T2
    q = q_squat;

% --- 段3：从蹲下 -> 站回原位 ---
elseif tau < T1 + T2 + T3
    u = (tau - (T1 + T2)) / T3;
    q = (1-u)*q_squat + u*q_stand;

% --- 结束后：保持站立 ---
else
    q = q_stand;
end
end

== matlab function Robot_Leg_Kneel/FR_climb/MATLAB Function1 ==
  data: t input; q output; mode_cmd input
function q = hip_FR_motion(t, mode_cmd)
%#codegen
% --- 右前腿 (Front Right) 髋关节 ---

T_squat_start = 5;
T_climb_start = 30;

% --- 阶段 0 & 1 ---
if (mode_cmd == 1) || (t < T_squat_start); q = 0; return; end
if t < T_climb_start
    tau = t - T_squat_start;
    q_stand = 0; q_squat = deg2rad(35);
    T1 = 3; T2 = 5; T3 = 3;
    if tau < T1; u=tau/T1; q=(1-u)*q_stand+u*q_squat;
    elseif tau < T1+T2; q=q_squat;
    elseif tau < T1+T2+T3; u=(tau-(T1+T2))/T3; q=(1-u)*q_squat+u*q_stand;
    else; q=q_stand; end
    return;
end

% ==========================================
% 阶段 2: 锁轮爬台阶 (130s 开始)
% ==========================================
tau = t - T_climb_start;
q_neutral = 0;
    q_fwd     = deg2rad(-5);
    
    % [130-132] 等待左前腿
    if tau < 4.0
        q = q_neutral;

    % [132-134] 第二步：抬腿迈向前方
    elseif tau < 8.0
        dt = tau - 4.0;
        u = dt / 4.0;
        q = (1-u)*q_neutral + u*q_fwd;
        
    % [134-138] 全身前移 (Body Shift)
    % 同样用力往回拉
    elseif tau < 12.0
        dt = tau - 8.0;
        u = dt / 6.0;
        u_smooth = 0.5 * (1 - cos(u * pi));
        q = (1-u_smooth)*q_fwd + u_smooth*q_neutral;
        
    else
        q = q_neutral;
    end
end

== matlab function Robot_Leg_Kneel/FR_climb/MATLAB Function4 ==
  data: t input; q output; mode_cmd input
function q = knee_FR_motion(t, mode_cmd)
%#codegen
% --- 右前腿 (Front Right) 膝关节 ---

T_squat_start = 5;
T_climb_start = 30;

% --- 阶段 0 & 1 ---
if (mode_cmd == 1) || (t < T_squat_start); q = 0; return; end
if t < T_climb_start
    tau = t - T_squat_start;
    q_stand = 0; q_squat = -deg2rad(70);
    T1 = 3; T2 = 5; T3 = 3;
    if tau < T1; u=tau/T1; q=(1-u)*q_stand+u*q_squat;
    elseif tau < T1+T2; q=q_squat;
    elseif tau < T1+T2+T3; u=(tau-(T1+T2))/T3; q=(1-u)*q_squat+u*q_stand;
    else; q=q_stand; end
    return;
end

% ==========================================
% 阶段 2: 锁轮爬台阶 (130s 开始)
% ==========================================
tau = t - T_climb_start;

q_stand = deg2rad(0);
    q_lift  = deg2rad(-20);

    % [130-132] 等待
    if tau < 4.0
        q = q_stand;
        
    % [132-134] 抬腿迈步
    elseif tau < 8.0
        dt = tau - 4.0;
        u = dt / 4.0;
        lift_scale = sin(u * pi);
        q = q_stand + lift_scale * (q_lift - q_stand);
        
    else
        q = q_stand;
    end
end

== matlab function Robot_Leg_Kneel/RL_climb/MATLAB Function2 ==
  data: t input; q output; mode_cmd input
function q = hip_RL_motion(t, mode_cmd)
%#codegen
% --- 左后腿 (Rear Left) 髋关节 ---
% 策略：锁轮爬行。先蹬地推身体，再收腿上台阶。

T_squat_start = 5;
T_climb_start = 30; 

% --- 阶段 0: 轮式/未开始 ---
if (mode_cmd == 1) || (t < T_squat_start); q = 0; return; end

% --- 阶段 1: 原地蹲起测试 (保持不变) ---
if t < T_climb_start
    tau = t - T_squat_start;
    q_stand = 0; q_squat = deg2rad(35);
    T1 = 3; T2 = 5; T3 = 3;
    if tau < T1; u=tau/T1; q=(1-u)*q_stand+u*q_squat;
    elseif tau < T1+T2; q=q_squat;
    elseif tau < T1+T2+T3; u=(tau-(T1+T2))/T3; q=(1-u)*q_squat+u*q_stand;
    else; q=q_stand;
    end
    return;
end

% ==========================================
% 阶段 2: 锁轮爬台阶 (130s 开始)
% ==========================================
tau = t - T_climb_start;
q_neutral = 0;
    q_push    = deg2rad(15); % 向后蹬的角度
    
    % [130-134] 前腿迈步时，后腿保持不动作为支撑
    if tau < 4.0
        q = q_neutral;
        
    % [134-138] 全身前移 (Body Shift)
    % 关键：前腿在拉，后腿要负责"推"！(从0变到+15)
    elseif tau < 8.0
        dt = tau - 4.0;
        u = dt / 4.0;
        u_smooth = 0.5 * (1 - cos(u * pi));
        q = (1-u_smooth)*q_neutral + u_smooth*q_push;
        
    % [138-140] 第四步：抬腿收回 (Swing Forward)
    % 从"后蹬"状态(+15) 抬起来回到 "中立"(0)
    elseif tau < 10.0
        dt = tau - 8.0;
        u = dt / 2.0;
        q = (1-u)*q_push + u*q_neutral;
        
    else
        q = q_neutral;
    end
end

== matlab function Robot_Leg_Kneel/RL_climb/MATLAB Function3 ==
  data: t input; q output; mode_cmd input
function q = knee_RL_motion(t, mode_cmd)
%#codegen
% --- 左后腿 (Rear Left) 膝关节 ---

T_squat_start = 5;
T_climb_start = 30;

% --- 阶段 0 & 1 (省略，保持不变) ---
if (mode_cmd == 1) || (t < T_squat_start); q = 0; return; end
if t < T_climb_start
    tau = t - T_squat_start;
    q_stand = 0; q_squat = -deg2rad(70);
    T1 = 3; T2 = 5; T3 = 3;
    if tau < T1; u=tau/T1; q=(1-u)*q_stand+u*q_squat;
    elseif tau < T1+T2; q=q_squat;
    elseif tau < T1+T2+T3; u=(tau-(T1+T2))/T3; q=(1-u)*q_squat+u*q_stand;
    else; q=q_stand;
    end
    return;
end

% ==========================================
% 阶段 2: 锁轮爬台阶 (130s 开始)
% ==========================================
tau = t - T_climb_start;

q_stand = deg2rad(0);
    q_lift  = deg2rad(-20);
    
    % [130-138] 支撑 + 推地
    if tau < 8.0
        q = q_stand;
        
    % [138-140] 抬腿收回
    elseif tau < 10.0
        dt = tau - 8.0;
        u = dt / 2.0;
        lift_scale = sin(u * pi);
        q = q_stand + lift_scale * (q_lift - q_stand);
        
    else
        q = q_stand;
    end
end

== matlab function Robot_Leg_Kneel/RR_climb/MATLAB Function2 ==
  data: t input; q output; mode_cmd input
function q = hip_RR_motion(t, mode_cmd)
%#codegen
% --- 右后腿 (Rear Right) 髋关节 ---

T_squat_start = 5;
T_climb_start = 30; 

if (mode_cmd == 1) || (t < T_squat_start); q = 0; return; end
% ... (省略蹲起阶段，请复制上面的) ...
if t < T_climb_start
    tau = t - T_squat_start;
    q_stand = 0; q_squat = deg2rad(35);
    T1 = 3; T2 = 5; T3 = 3;
    if tau < T1; u=tau/T1; q=(1-u)*q_stand+u*q_squat;
    elseif tau < T1+T2; q=q_squat;
    elseif tau < T1+T2+T3; u=(tau-(T1+T2))/T3; q=(1-u)*q_squat+u*q_stand;
    else; q=q_stand;
    end
    return;
end


tau = t - T_climb_start;

q_neutral = 0;
    q_push    = deg2rad(15);
    
    % [130-134] 支撑
    if tau < 4.0
        q = q_neutral;
        
    % [134-138] 推地 (Body Shift)
    elseif tau < 8.0
        dt = tau - 4.0;
        u = dt / 4.0;
        u_smooth = 0.5 * (1 - cos(u * pi));
        q = (1-u_smooth)*q_neutral + u_smooth*q_push;
        
    % [138-140] 等待左后腿收完 (保持推地状态支撑)
    elseif tau < 10.0
        q = q_push;

    % [140-142] 第五步：抬腿收回
    elseif tau < 12.0
        dt = tau - 10.0;
        u = dt / 2.0;
        q = (1-u)*q_push + u*q_neutral;
        
    else
        q = q_neutral;
    end
end

== matlab function Robot_Leg_Kneel/RR_climb/MATLAB Function4 ==
  data: t input; q output; mode_cmd input
function q = knee_RR_motion(t, mode_cmd)
%#codegen
% --- 右后腿 (Rear Right) 膝关节 ---

T_squat_start = 5;
T_climb_start = 30;

if (mode_cmd == 1) || (t < T_squat_start); q = 0; return; end
% ... (省略蹲起阶段) ...
if t < T_climb_start
    tau = t - T_squat_start;
    q_stand = 0; q_squat = -deg2rad(70);
    T1 = 3; T2 = 5; T3 = 3;
    if tau < T1; u=tau/T1; q=(1-u)*q_stand+u*q_squat;
    elseif tau < T1+T2; q=q_squat;
    elseif tau < T1+T2+T3; u=(tau-(T1+T2))/T3; q=(1-u)*q_squat+u*q_stand;
    else; q=q_stand;
    end
    return;
end


tau = t - T_climb_start;

q_stand = deg2rad(0);
    q_lift  = deg2rad(-20);

    % [130-140] 支撑 + 推地
    if tau < 10.0
        q = q_stand;
        
    % [140-142] 抬腿收回
    elseif tau < 12.0
        dt = tau - 10.0;
        u = dt / 2.0;
        lift_scale = sin(u * pi);
        q = q_stand + lift_scale * (q_lift - q_stand);
        
    else
        q = q_stand;
    end
end

== matlab function Robot_Leg_Kneel/RL/MATLAB Function5 ==
  settings: updateMethod=DISCRETE
  data: mode_cmd input; tau output; q input; dq input
function tau = WheelLockPD(mode_cmd, q, dq)
%#codegen
% mode_cmd: 0=Walk (lock wheel), 1=Wheeled (don't lock wheel)
% q, dq measurements from the wheel axle Revolute Joint
% Braking PD parameters (tunable)
Kp = 50.0;     % Braking stiffness, smaller to avoid being too rigid
Kd =  5.0;     % Damping
tau_lim = 150.0;  % Maximum braking torque for the wheel
% Lock only in walk mode
lock = (mode_cmd == 0);
persistent q_hold last_lock
if isempty(q_hold),    q_hold    = q;     end
if isempty(last_lock), last_lock = false; end
% The moment it switches from "unlocked" to "locked", remember the current angle
if (~last_lock) && lock
    q_hold = q;
end
last_lock = lock;
if lock
    % Lock wheel: treat q_hold as the target angle
    q_ref  = q_hold;
    dq_ref = 0.0;
    tau = Kp*(q_ref - q) + Kd*(dq_ref - dq);
else
    % Wheeled mode: do not apply brake
    tau = 0.0;
end
% Torque saturation
if tau >  tau_lim, tau =  tau_lim; end
if tau < -tau_lim, tau = -tau_lim; end
end

== matlab function Robot_Leg_Kneel/RR/MATLAB Function5 ==
  settings: updateMethod=DISCRETE
  data: mode_cmd input; tau output; q input; dq input
function tau = WheelLockPD(mode_cmd, q, dq)
%#codegen
% mode_cmd: 0=Walk (lock wheel), 1=Wheeled (don't lock wheel)
% q, dq measurements from the wheel axle Revolute Joint
% Braking PD parameters (tunable)
Kp = 50.0;     % Braking stiffness, smaller to avoid being too rigid
Kd =  5.0;     % Damping
tau_lim = 150.0;  % Maximum braking torque for the wheel
% Lock only in walk mode
lock = (mode_cmd == 0);
persistent q_hold last_lock
if isempty(q_hold),    q_hold    = q;     end
if isempty(last_lock), last_lock = false; end
% The moment it switches from "unlocked" to "locked", remember the current angle
if (~last_lock) && lock
    q_hold = q;
end
last_lock = lock;
if lock
    % Lock wheel: treat q_hold as the target angle
    q_ref  = q_hold;
    dq_ref = 0.0;
    tau = Kp*(q_ref - q) + Kd*(dq_ref - dq);
else
    % Wheeled mode: do not apply brake
    tau = 0.0;
end
% Torque saturation
if tau >  tau_lim, tau =  tau_lim; end
if tau < -tau_lim, tau = -tau_lim; end
end

== matlab function Robot_Leg_Kneel/RR/MATLAB Function ==
  data: mode_cmd input; alpha input; tau output; q input; dq input; q_cmd input; is_locked output; q_ref output
function [tau, is_locked, q_ref] = LockJointPD(mode_cmd, alpha, q, dq, q_cmd)
%#codegen
% mode_cmd: 0=Walk(folloew q_cmd), 1=Wheel(lock the present angle )
% alpha   : [0,1] flatten faktor(TransferFcnoutput)，0=walk, 1=leg locked
% q,dq    : joint angle/angular velocity
% q_cmd   : walking/standing angle(rad)

Kp = 1200.0;   % start value
Kd =   20.0;
tau_lim = 300.0;

m = uint8(mode_cmd ~= 0);     % uint8(0/1)
a = double(alpha);

persistent q_hold last_mode
if isempty(q_hold),    q_hold    = q;        end   % double
if isempty(last_mode), last_mode = uint8(0); end   % uint8

% step: 0->1 
if (last_mode == uint8(0)) && (m ~= uint8(0))
    q_hold = q;
end
last_mode = m;

% reference angle
q_ref  = a*q_hold + (1-a)*q_cmd;
dq_ref = 0.0;

% PD
tau = Kp*(q_ref - q) + Kd*(dq_ref - dq);

% 
tau = max(min(tau, tau_lim), -tau_lim);

% 
is_locked = (a > 0.5);     % 
end

== matlab function Robot_Leg_Kneel/RR1/MATLAB Function ==
  data: mode_cmd input; alpha input; tau output; q input; dq input; q_cmd input; is_locked output; q_ref output
function [tau, is_locked, q_ref] = LockJointPD(mode_cmd, alpha, q, dq, q_cmd)
%#codegen
% mode_cmd: 0=Walk(folloew q_cmd), 1=Wheel(lock the present angle )
% alpha   : [0,1] flatten faktor(TransferFcnoutput)，0=walk, 1=leg locked
% q,dq    : joint angle/angular velocity
% q_cmd   : walking/standing angle(rad)

Kp = 1200.0;   % start value
Kd =   20.0;
tau_lim = 300.0;

m = uint8(mode_cmd ~= 0);     % uint8(0/1)
a = double(alpha);

persistent q_hold last_mode
if isempty(q_hold),    q_hold    = q;        end   % double
if isempty(last_mode), last_mode = uint8(0); end   % uint8

% step: 0->1 
if (last_mode == uint8(0)) && (m ~= uint8(0))
    q_hold = q;
end
last_mode = m;

% reference angle
q_ref  = a*q_hold + (1-a)*q_cmd;
dq_ref = 0.0;

% PD
tau = Kp*(q_ref - q) + Kd*(dq_ref - dq);

% 
tau = max(min(tau, tau_lim), -tau_lim);

% 
is_locked = (a > 0.5);     % 
end

== matlab function Robot_Leg_Kneel/RR1/MATLAB Function1 ==
  data: mode_cmd input; alpha input; tau output; q input; dq input; q_cmd input; is_locked output; q_ref output
function [tau, is_locked, q_ref] = LockJointPD(mode_cmd, alpha, q, dq, q_cmd)
%#codegen
% mode_cmd: 0=Walk (track q_cmd), 1=Wheeled (lock current angle)
% alpha   : [0,1] smoothing factor (TransferFcn output), 0=fully walking, 1=fully locked
% q,dq    : joint angle/angular velocity
% q_cmd   : walk/stand target angle (radians)
Kp = 1200.0;   % Starting value, tune per joint
Kd =   20.0;
tau_lim = 300.0;
m = uint8(mode_cmd ~= 0);     % Standardize to uint8(0/1)
a = double(alpha);
persistent q_hold last_mode
if isempty(q_hold),    q_hold    = q;        end   % double
if isempty(last_mode), last_mode = uint8(0); end   % uint8
% Rising edge: 0->1, latch current angle
if (last_mode == uint8(0)) && (m ~= uint8(0))
    q_hold = q;
end
last_mode = m;
% Reference angle: interpolate between "hold angle" and "target angle"
q_ref  = a*q_hold + (1-a)*q_cmd;
dq_ref = 0.0;
% PD
tau = Kp*(q_ref - q) + Kd*(dq_ref - dq);
% Saturation
tau = max(min(tau, tau_lim), -tau_lim);
% Debug flag: is leg lock dominant
is_locked = (a > 0.5);     % Can also output m==1
end

== matlab function Robot_Leg_Kneel/RL1/MATLAB Function ==
  data: mode_cmd input; alpha input; tau output; q input; dq input; q_cmd input; is_locked output; q_ref output
function [tau, is_locked, q_ref] = LockJointPD(mode_cmd, alpha, q, dq, q_cmd)
%#codegen
% mode_cmd: 0=Walk (track q_cmd), 1=Wheeled (lock current angle)
% alpha   : [0,1] smoothing factor (TransferFcn output), 0=fully walking, 1=fully locked
% q,dq    : joint angle/angular velocity
% q_cmd   : walk/stand target angle (radians)
Kp = 1200.0;   % Starting value, tune per joint
Kd =   20.0;
tau_lim = 300.0;
m = uint8(mode_cmd ~= 0);     % Standardize to uint8(0/1)
a = double(alpha);
persistent q_hold last_mode
if isempty(q_hold),    q_hold    = q;        end   % double
if isempty(last_mode), last_mode = uint8(0); end   % uint8
% Rising edge: 0->1, latch current angle
if (last_mode == uint8(0)) && (m ~= uint8(0))
    q_hold = q;
end
last_mode = m;
% Reference angle: interpolate between "hold angle" and "target angle"
q_ref  = a*q_hold + (1-a)*q_cmd;
dq_ref = 0.0;
% PD
tau = Kp*(q_ref - q) + Kd*(dq_ref - dq);
% Saturation
tau = max(min(tau, tau_lim), -tau_lim);
% Debug flag: is leg lock dominant
is_locked = (a > 0.5);     % Can also output m==1
end

== matlab function Robot_Leg_Kneel/RL1/MATLAB Function1 ==
  data: mode_cmd input; alpha input; tau output; q input; dq input; q_cmd input; is_locked output; q_ref output
function [tau, is_locked, q_ref] = LockJointPD(mode_cmd, alpha, q, dq, q_cmd)
%#codegen
% mode_cmd: 0=Walk (track q_cmd), 1=Wheeled (lock current angle)
% alpha   : [0,1] smoothing factor (TransferFcn output), 0=fully walking, 1=fully locked
% q,dq    : joint angle/angular velocity
% q_cmd   : walk/stand target angle (radians)
Kp = 1200.0;   % Starting value, tune per joint
Kd =   20.0;
tau_lim = 300.0;
m = uint8(mode_cmd ~= 0);     % Standardize to uint8(0/1)
a = double(alpha);
persistent q_hold last_mode
if isempty(q_hold),    q_hold    = q;        end   % double
if isempty(last_mode), last_mode = uint8(0); end   % uint8
% Rising edge: 0->1, latch current angle
if (last_mode == uint8(0)) && (m ~= uint8(0))
    q_hold = q;
end
last_mode = m;
% Reference angle: interpolate between "hold angle" and "target angle"
q_ref  = a*q_hold + (1-a)*q_cmd;
dq_ref = 0.0;
% PD
tau = Kp*(q_ref - q) + Kd*(dq_ref - dq);
% Saturation
tau = max(min(tau, tau_lim), -tau_lim);
% Debug flag: is leg lock dominant
is_locked = (a > 0.5);     % Can also output m==1
end
